simulink model "ECR3"  (Simulink 8.3)
settings: Solver=ode45  StartTime=0.0  StopTime=50  RelTol=1e-4
undefined symbols (not defined in the file or in its folder): Engine, Trans
libraries: simulink x2
settings Model: Creator=swami  LastModifiedBy=swami
settings SolverCC: ShapePreserveControl=EnableAll  ZeroCrossControl=EnableAll
settings DataIOCC: SignalLoggingSaveFormat=Dataset
settings DebuggingCC: UnderspecifiedInitializationDetection=Simplified  StateNameClashWarn=none
settings ModelReferenceCC: UpdateModelReferenceTargets=Force
settings GRTTargetCC: CombineOutputUpdateFcns=on  GRTInterface=off

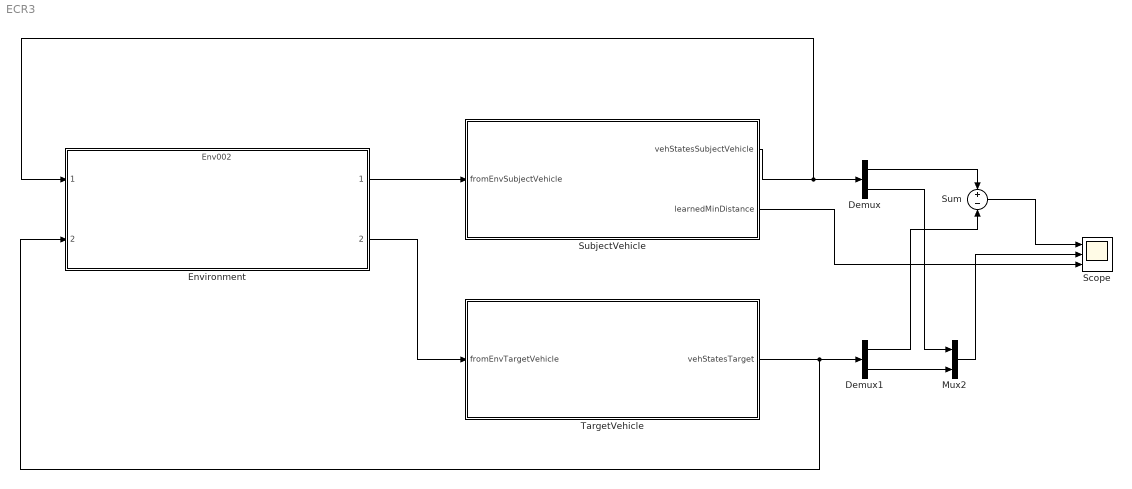
== system ECR3 ==
  Demux : Demux  Outputs=2
  Demux1 : Demux  Outputs=2
  Environment : ModelReference  ModelNameDialog=Env002.mdl  SimulationMode=Normal  Variant=on  OverrideUsingVariant=varObject1  ModelReferenceVersion=1.10  CopyOfModelName=Env002.mdl  DefaultDataLogging=on
      settings: AttributesFormatString=%<ActiveVariant>
  Mux2 : Mux  Inputs=2
  Scope : Scope  NumInputPorts=3
      settings: YMin=-5~-5~-5  YMax=5~5~5
  SubjectVehicle : Subsystem
  Sum : Sum  Inputs=+-
  TargetVehicle : Subsystem
  wires:
  Environment/1 -> SubjectVehicle/1(fromEnvSubjectVehicle)
  SubjectVehicle/1(vehStatesSubjectVehicle) -> Environment/1, Demux/1
  TargetVehicle/1(vehStatesTarget) -> Demux1/1, Environment/2
  Environment/2 -> TargetVehicle/1(fromEnvTargetVehicle)
  Demux/1 -> Sum/1
  Demux1/1 -> Sum/2
  Demux/2 -> Mux2/1
  Demux1/2 -> Mux2/2
  Mux2/1 -> Scope/2
  Sum/1 -> Scope/1
  SubjectVehicle/2(learnedMinDistance) -> Scope/3

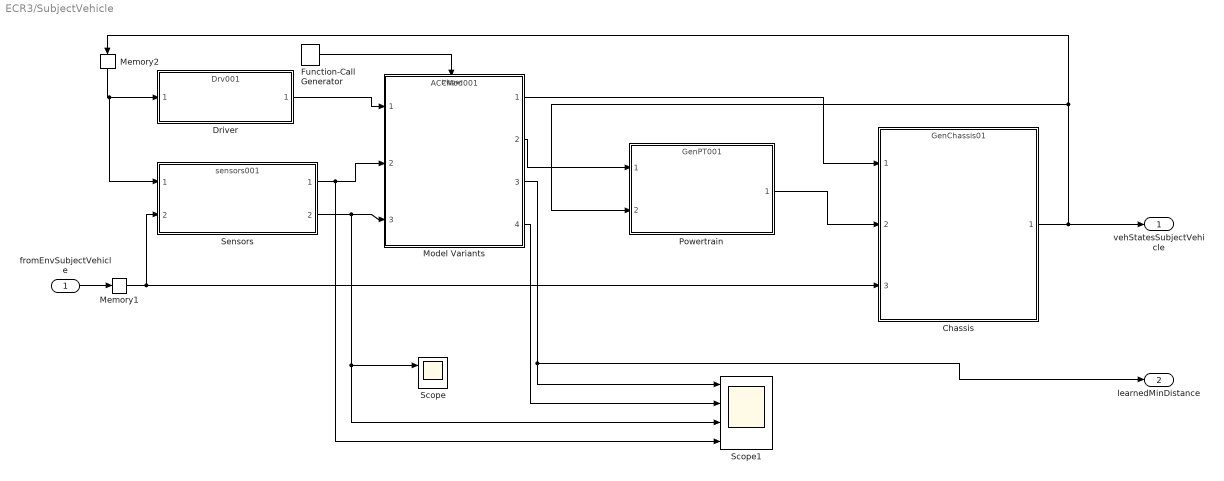
== system ECR3/SubjectVehicle ==
  fromEnvSubjectVehicle : Inport
  Chassis : ModelReference  ModelNameDialog=GenChassis01  ParameterArgumentNames=Chassis  ParameterArgumentValues=ChassisSubject  SimulationMode=Normal  Variant=on  ModelReferenceVersion=1.19  CopyOfModelName=GenChassis01  DefaultDataLogging=on
      settings: AttributesFormatString=%<ActiveVariant>
  Driver : ModelReference  ModelNameDialog=Drv001  ParameterArgumentNames=pDrv  ParameterArgumentValues=DrvSubject  SimulationMode=Normal  Variant=on  ModelReferenceVersion=1.20  CopyOfModelName=Drv001  DefaultDataLogging=on
      settings: AttributesFormatString=%<ActiveVariant>
  Function-Call Generator : simulink/Ports & Subsystems/Function-Call Generator  sample_time=0.1  numberOfIterations=1
  Memory1 : Memory
  Memory2 : Memory
  Model Variants : ModelReference  ModelNameDialog=ACCMod001.mdl  ParameterArgumentNames=pACC  ParameterArgumentValues=pACCMod  SimulationMode=Normal  Variant=on  OverrideUsingVariant=varObject1  ModelReferenceVersion=1.115  CopyOfModelName=ACCMod001.mdl  DefaultDataLogging=on  TriggerPortName=Trigger  TriggerPortTriggerType=function-call  TriggerPortStatesWhenEnabling=held
      settings: AttributesFormatString=%<ActiveVariant>
  Powertrain : ModelReference  ModelNameDialog=GenPT001  ParameterArgumentNames=Trans,Engine  ParameterArgumentValues=Trans,Engine  SimulationMode=Normal  Variant=on  ModelReferenceVersion=1.23  CopyOfModelName=GenPT001  DefaultDataLogging=on
      settings: AttributesFormatString=%<ActiveVariant>
  Scope : Scope  NumInputPorts=2
      settings: YMin=-5~-5  YMax=5~5
  Scope1 : Scope  NumInputPorts=4
      settings: TimeRange=50  YMin=-5~-5~-5~-5  YMax=5~5~5~5  SaveName=ScopeData2
  Sensors : ModelReference  ModelNameDialog=sensors001  SimulationMode=Normal  Variant=on  ModelReferenceVersion=1.18  CopyOfModelName=sensors001  DefaultDataLogging=on
      settings: AttributesFormatString=%<ActiveVariant>
  vehStatesSubjectVehicle : Outport
  learnedMinDistance : Outport  Port=2
  wires:
  Chassis/1 -> Powertrain/2, Memory2/1, vehStatesSubjectVehicle/1
  Model Variants/2 -> Powertrain/1
  Powertrain/1 -> Chassis/2
  Model Variants/1 -> Chassis/1
  Sensors/1 -> Model Variants/2, Scope1/4
  Sensors/2 -> Scope/1, Scope1/3, Model Variants/3
  Model Variants/3 -> learnedMinDistance/1, Scope1/1
  Model Variants/4 -> Scope1/2
  Driver/1 -> Model Variants/1
  Memory2/1 -> Sensors/1, Driver/1
  fromEnvSubjectVehicle/1 -> Memory1/1
  Memory1/1 -> Sensors/2, Chassis/3
  Function-Call Generator/1 -> Model Variants/Trigger

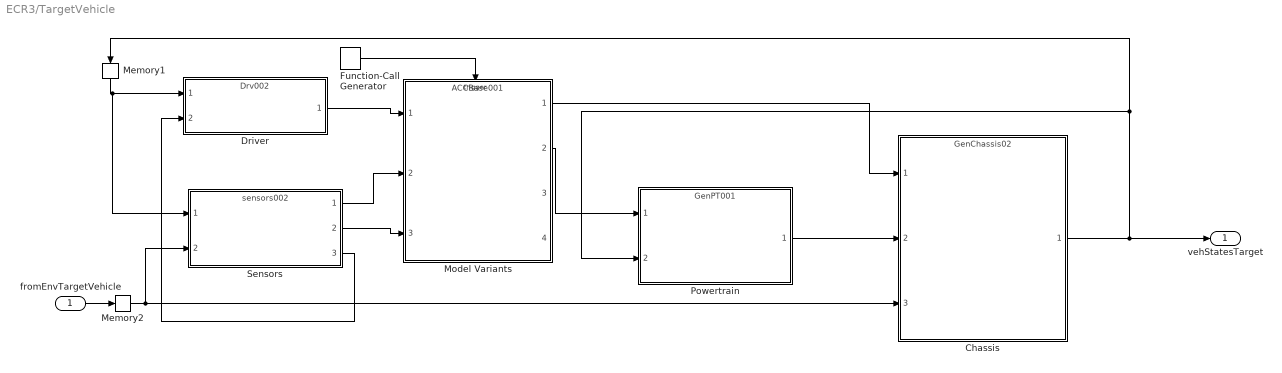
== system ECR3/TargetVehicle ==
  fromEnvTargetVehicle : Inport
  Chassis : ModelReference  ModelNameDialog=GenChassis02.mdl  ParameterArgumentNames=Chassis  ParameterArgumentValues=ChassisTarget  SimulationMode=Normal  Variant=on  OverrideUsingVariant=varObject1  ModelReferenceVersion=1.19  CopyOfModelName=GenChassis02.mdl  DefaultDataLogging=on
      settings: AttributesFormatString=%<ActiveVariant>
  Driver : ModelReference  ModelNameDialog=Drv002.mdl  ParameterArgumentNames=pDrv  ParameterArgumentValues=DrvTarget  SimulationMode=Normal  Variant=on  OverrideUsingVariant=varObject1  ModelReferenceVersion=1.48  CopyOfModelName=Drv002.mdl  DefaultDataLogging=on
      settings: AttributesFormatString=%<ActiveVariant>
  Function-Call Generator : simulink/Ports & Subsystems/Function-Call Generator  sample_time=0.1  numberOfIterations=1
  Memory1 : Memory
  Memory2 : Memory
  Model Variants : ModelReference  ModelNameDialog=ACCBase001  ParameterArgumentNames=pACC  ParameterArgumentValues=pACCBase  SimulationMode=Normal  Variant=on  ModelReferenceVersion=1.92  CopyOfModelName=ACCBase001  DefaultDataLogging=on  TriggerPortName=Trigger  TriggerPortTriggerType=function-call  TriggerPortStatesWhenEnabling=held
      settings: AttributesFormatString=%<ActiveVariant>
  Powertrain : ModelReference  ModelNameDialog=GenPT001  ParameterArgumentNames=Trans,Engine  ParameterArgumentValues=Trans,Engine  SimulationMode=Normal  Variant=on  ModelReferenceVersion=1.23  CopyOfModelName=GenPT001  DefaultDataLogging=on
      settings: AttributesFormatString=%<ActiveVariant>
  Sensors : ModelReference  ModelNameDialog=sensors002.mdl  SimulationMode=Normal  Variant=on  OverrideUsingVariant=varObject1  ModelReferenceVersion=1.19  CopyOfModelName=sensors002.mdl  DefaultDataLogging=on
      settings: AttributesFormatString=%<ActiveVariant>
  vehStatesTarget : Outport
  wires:
  Sensors/2 -> Model Variants/3
  Sensors/1 -> Model Variants/2
  Driver/1 -> Model Variants/1
  Model Variants/1 -> Chassis/1
  Powertrain/1 -> Chassis/2
  Model Variants/2 -> Powertrain/1
  fromEnvTargetVehicle/1 -> Memory2/1
  Chassis/1 -> vehStatesTarget/1, Memory1/1, Powertrain/2
  Sensors/3 -> Driver/2
  Memory1/1 -> Sensors/1, Driver/1
  Memory2/1 -> Sensors/2, Chassis/3
  Function-Call Generator/1 -> Model Variants/Trigger
